simulink model "NeuromuscularModel2D"  (R2019b)
settings: Solver=ode15s  StartTime=0.0  StopTime=30  MaxStep=.01  RelTol=1e-4  AbsTol=1e-6  EnableMultiTasking=on
values from neighbouring files (symbols this model uses):
  dt_visual = 1/50    (= 0.02)    [evaluateCost.m]    (also in optimize.m = 0.0333333333333; setVars.m = 0.0333333333333)
  initialTargetAngle = 70*pi/180    (= 1.2217304764)    [ControlParams.m]    (also in setInit.m)
  LongDelay = 0.020/2    (= 0.01)    [ControlParams.m]
  LongLoopDelay = 0.030    (= 0.03)    [ControlParams.m]
  MidDelay = 0.010/2    (= 0.005)    [ControlParams.m]
  N = {S.name}    [mergeCompareEnergyCosts.m]
  PreStimBFSHst = 0.02    [ControlParams.m]    (also in assignGainsSagittal.m = GainsSagittal(51))
  PreStimBFSHsw = 0.02    [ControlParams.m]    (also in assignGainsSagittal.m = GainsSagittal(60))
  PreStimGASst = 0.01    [ControlParams.m]    (also in assignGainsSagittal.m = GainsSagittal(52))
  PreStimGASsw = 0.01    [ControlParams.m]    (also in assignGainsSagittal.m = GainsSagittal(61))
  PreStimGLUst = 0.05    [ControlParams.m]    (also in assignGainsSagittal.m = GainsSagittal(47))
  PreStimGLUsw = 0.01    [ControlParams.m]    (also in assignGainsSagittal.m = GainsSagittal(56))
  PreStimHAMst = 0.05    [ControlParams.m]    (also in assignGainsSagittal.m = GainsSagittal(48))
  PreStimHAMsw = 0.01    [ControlParams.m]    (also in assignGainsSagittal.m = GainsSagittal(57))
  PreStimHFLst = 0.05    [ControlParams.m]    (also in assignGainsSagittal.m = GainsSagittal(46))
  PreStimHFLsw = 0.01    [ControlParams.m]    (also in assignGainsSagittal.m = GainsSagittal(55))
  PreStimRFst = 0.01    [ControlParams.m]    (also in assignGainsSagittal.m = GainsSagittal(49))
  PreStimRFsw = 0.01    [ControlParams.m]    (also in assignGainsSagittal.m = GainsSagittal(58))
  PreStimSOLst = 0.01    [ControlParams.m]    (also in assignGainsSagittal.m = GainsSagittal(53))
  PreStimSOLsw = 0.01    [ControlParams.m]    (also in assignGainsSagittal.m = GainsSagittal(62))
  PreStimTAst = 0.01    [ControlParams.m]    (also in assignGainsSagittal.m = GainsSagittal(54))
  PreStimTAsw = 0.01    [ControlParams.m]    (also in assignGainsSagittal.m = GainsSagittal(63))
  PreStimVASst = 0.08    [ControlParams.m]    (also in assignGainsSagittal.m = GainsSagittal(50))
  PreStimVASsw = 0.01    [ControlParams.m]    (also in assignGainsSagittal.m = GainsSagittal(59))
  ShortDelay = 0.005/2    (= 0.0025)    [ControlParams.m]
  termination_height = 0.5    [ControlParams.m]
  X = ~cellfun('isempty',strfind(N,'compareEnergyCost'))    [mergeCompareEnergyCosts.m]
undefined symbols (not defined in the file or in its folder): g, hatLeftHipToCenterDistWidth, hatLeftHipToCG, initialTargetAngleR, magnitude, obstacle_depth, obstacle_height, obstacle_width, obstacle_x, PreStimHABst, PreStimHABsw, PreStimHADst, PreStimHADsw, thetaHATref, Y, Z
libraries: NeuroMuscularLibrary x96, sm_lib x20, nesl_utility x19, simulink x3
(part 3 of 3)

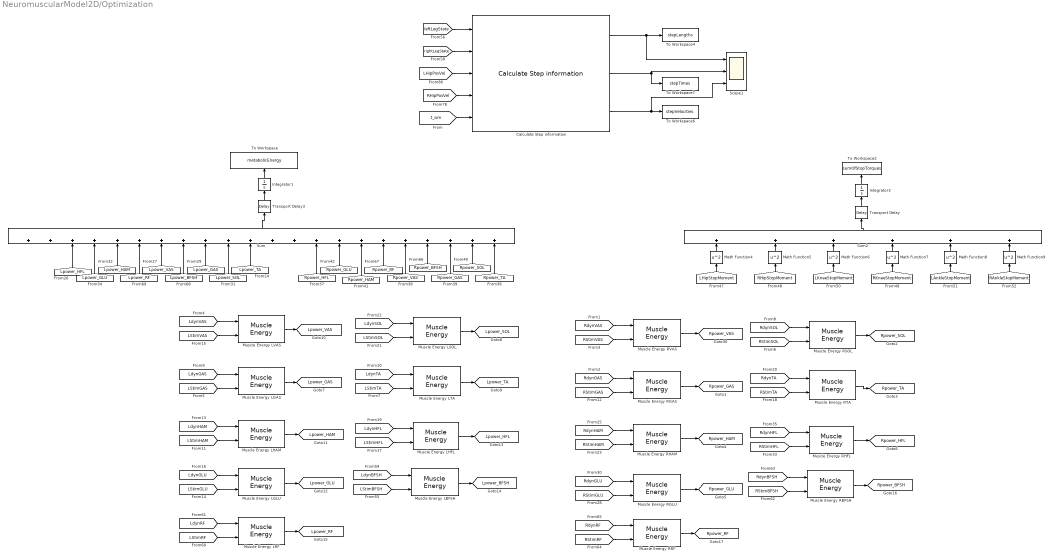
== system NeuromuscularModel2D/Optimization ==
  Calculate Step information : NeuroMuscularLibrary/Calculate Step information  SystemSampleTime=-1  Latency=0  AutoFrameSizeCalculation=off
  Integrator1 : Integrator
  Integrator3 : Integrator
  Math Function{4..9} (6 alike) : Math  Operator=square  SaturateOnIntegerOverflow=on
  Muscle Energy LBFSH : NeuroMuscularLibrary/Muscle Energy  lopt=loptBFSH  FT=FT_BFSH  Fmax=FmaxBFSH  vmax=vmaxBFSH
  Muscle Energy LGAS : NeuroMuscularLibrary/Muscle Energy  lopt=loptGAS  FT=FT_GAS  Fmax=FmaxGAS  vmax=vmaxGAS
  Muscle Energy LGLU : NeuroMuscularLibrary/Muscle Energy  lopt=loptGLU  FT=FT_GLU  Fmax=FmaxGLU  vmax=vmaxGLU
  Muscle Energy LHAM : NeuroMuscularLibrary/Muscle Energy  lopt=loptHAM  FT=FT_HAM  Fmax=FmaxHAM  vmax=vmaxHAM
  Muscle Energy LHFL : NeuroMuscularLibrary/Muscle Energy  lopt=loptHFL  FT=FT_HFL  Fmax=FmaxHFL  vmax=vmaxHFL
  Muscle Energy LRF : NeuroMuscularLibrary/Muscle Energy  lopt=loptRF  FT=FT_RF  Fmax=FmaxRF  vmax=vmaxRF
  Muscle Energy LSOL : NeuroMuscularLibrary/Muscle Energy  lopt=loptSOL  FT=FT_SOL  Fmax=FmaxSOL  vmax=vmaxSOL
  Muscle Energy LTA : NeuroMuscularLibrary/Muscle Energy  lopt=loptTA  FT=FT_TA  Fmax=FmaxTA  vmax=vmaxTA
  Muscle Energy LVAS : NeuroMuscularLibrary/Muscle Energy  lopt=loptVAS  FT=FT_VAS  Fmax=FmaxVAS  vmax=vmaxVAS
  Muscle Energy RBFSH : NeuroMuscularLibrary/Muscle Energy  lopt=loptBFSH  FT=FT_BFSH  Fmax=FmaxBFSH  vmax=vmaxBFSH
  Muscle Energy RGAS : NeuroMuscularLibrary/Muscle Energy  lopt=loptGAS  FT=FT_GAS  Fmax=FmaxGAS  vmax=vmaxGAS
  Muscle Energy RGLU : NeuroMuscularLibrary/Muscle Energy  lopt=loptGLU  FT=FT_GLU  Fmax=FmaxGLU  vmax=vmaxGLU
  Muscle Energy RHAM : NeuroMuscularLibrary/Muscle Energy  lopt=loptHAM  FT=FT_HAM  Fmax=FmaxHAM  vmax=vmaxHAM
  Muscle Energy RHFL : NeuroMuscularLibrary/Muscle Energy  lopt=loptHFL  FT=FT_HFL  Fmax=FmaxHFL  vmax=vmaxHFL
  Muscle Energy RRF : NeuroMuscularLibrary/Muscle Energy  lopt=loptRF  FT=FT_RF  Fmax=FmaxRF  vmax=vmaxRF
  Muscle Energy RSOL : NeuroMuscularLibrary/Muscle Energy  lopt=loptSOL  FT=FT_SOL  Fmax=FmaxSOL  vmax=vmaxSOL
  Muscle Energy RTA : NeuroMuscularLibrary/Muscle Energy  lopt=loptTA  FT=FT_TA  Fmax=FmaxTA  vmax=vmaxTA
  Muscle Energy RVAS : NeuroMuscularLibrary/Muscle Energy  lopt=loptVAS  FT=FT_VAS  Fmax=FmaxVAS  vmax=vmaxVAS
  Scope1 : Scope  NumInputPorts=3
  Sum : Sum  Inputs=++++++++++++++++++++++
  Sum2 : Sum  Inputs=++++++
  To Workspace : ToWorkspace  VariableName=metabolicEnergy  SampleTime=-1
      settings: MaxDataPoints=1
  To Workspace2 : ToWorkspace  VariableName=sumOfStopTorques  SampleTime=-1
      settings: MaxDataPoints=1
  To Workspace4 : ToWorkspace  VariableName=stepLengths  SampleTime=-1
  To Workspace6 : ToWorkspace  VariableName=stepVelocities  SampleTime=-1
  To Workspace7 : ToWorkspace  VariableName=stepTimes  SampleTime=-1
  Transport Delay : TransportDelay  DelayTime=3  BufferSize=24576
  Transport Delay3 : TransportDelay  DelayTime=3  BufferSize=24576
  tag scope: Lpower_BFSH=global, Lpower_GAS=global, Lpower_GLU=global, Lpower_HAM=global, Lpower_HFL=global, Lpower_RF=global, Lpower_SOL=global, Lpower_TA=global, Lpower_VAS=global, Rpower_BFSH=global, Rpower_GAS=global, Rpower_GLU=global, Rpower_HAM=global, Rpower_HFL=global, Rpower_RF=global, Rpower_SOL=global, Rpower_TA=global, Rpower_VAS=global
  wires:
  [RdynSOL] -> Muscle Energy RSOL/1
  [RStimSOL] -> Muscle Energy RSOL/2
  [RStimVAS] -> Muscle Energy RVAS/2
  [RStimGAS] -> Muscle Energy RGAS/2
  Muscle Energy RVAS/1 -> [Rpower_VAS]
  Muscle Energy RGAS/1 -> [Rpower_GAS]
  Muscle Energy RSOL/1 -> [Rpower_SOL]
  Muscle Energy RTA/1 -> [Rpower_TA]
  [RdynTA] -> Muscle Energy RTA/1
  [RStimTA] -> Muscle Energy RTA/2
  [RdynHAM] -> Muscle Energy RHAM/1
  [RStimHAM] -> Muscle Energy RHAM/2
  [RdynGLU] -> Muscle Energy RGLU/1
  [RStimGLU] -> Muscle Energy RGLU/2
  [RdynHFL] -> Muscle Energy RHFL/1
  [RStimHFL] -> Muscle Energy RHFL/2
  Muscle Energy RHAM/1 -> [Rpower_HAM]
  Muscle Energy RGLU/1 -> [Rpower_GLU]
  Muscle Energy RHFL/1 -> [Rpower_HFL]
  [Lpower_VAS] -> Sum/7
  [Lpower_RF] -> Sum/6
  [Lpower_HAM] -> Sum/5
  [Lpower_GLU] -> Sum/4
  [Lpower_HFL] -> Sum/3
  [RdynGAS] -> Muscle Energy RGAS/1
  [RdynVAS] -> Muscle Energy RVAS/1
  [LdynSOL] -> Muscle Energy LSOL/1
  [LStimSOL] -> Muscle Energy LSOL/2
  [LStimVAS] -> Muscle Energy LVAS/2
  [LStimGAS] -> Muscle Energy LGAS/2
  Muscle Energy LVAS/1 -> [Lpower_VAS]
  Muscle Energy LGAS/1 -> [Lpower_GAS]
  Muscle Energy LSOL/1 -> [Lpower_SOL]
  Muscle Energy LTA/1 -> [Lpower_TA]
  [LdynTA] -> Muscle Energy LTA/1
  [LStimTA] -> Muscle Energy LTA/2
  [LdynHAM] -> Muscle Energy LHAM/1
  [LStimHAM] -> Muscle Energy LHAM/2
  [LdynGLU] -> Muscle Energy LGLU/1
  [LStimGLU] -> Muscle Energy LGLU/2
  [LdynHFL] -> Muscle Energy LHFL/1
  [LStimHFL] -> Muscle Energy LHFL/2
  Muscle Energy LHAM/1 -> [Lpower_HAM]
  Muscle Energy LGLU/1 -> [Lpower_GLU]
  Muscle Energy LHFL/1 -> [Lpower_HFL]
  [LdynGAS] -> Muscle Energy LGAS/1
  [LdynVAS] -> Muscle Energy LVAS/1
  [Lpower_SOL] -> Sum/10
  [Rpower_HAM] -> Sum/16
  [Rpower_GLU] -> Sum/15
  [Rpower_HFL] -> Sum/14
  [Lpower_TA] -> Sum/11
  Integrator1/1 -> To Workspace/1
  Sum/1 -> Transport Delay3/1
  Integrator3/1 -> To Workspace2/1
  Math Function4/1 -> Sum2/1
  [LHipStopMoment] -> Math Function4/1
  Math Function5/1 -> Sum2/2
  [RHipStopMoment] -> Math Function5/1
  Math Function6/1 -> Sum2/3
  Math Function7/1 -> Sum2/4
  [LKneeStopMoment] -> Math Function6/1
  [RKneeStopMoment] -> Math Function7/1
  [LAnkleStopMoment] -> Math Function8/1
  Math Function8/1 -> Sum2/5
  [RAnkleStopMoment] -> Math Function9/1
  Math Function9/1 -> Sum2/6
  Transport Delay/1 -> Integrator3/1
  Sum2/1 -> Transport Delay/1
  Transport Delay3/1 -> Integrator1/1
  [rightLegState] -> Calculate Step information/2
  Calculate Step information/1 -> Scope1/1, To Workspace4/1
  Calculate Step information/3 -> To Workspace6/1, Scope1/3
  Calculate Step information/2 -> To Workspace7/1, Scope1/2
  [leftLegState] -> Calculate Step information/1
  [t_sim] -> Calculate Step information/5
  Muscle Energy LBFSH/1 -> [Lpower_BFSH]
  [LStimBFSH] -> Muscle Energy LBFSH/2
  [LdynBFSH] -> Muscle Energy LBFSH/1
  [LdynRF] -> Muscle Energy LRF/1
  [LStimRF] -> Muscle Energy LRF/2
  Muscle Energy LRF/1 -> [Lpower_RF]
  Muscle Energy RRF/1 -> [Rpower_RF]
  [RdynRF] -> Muscle Energy RRF/1
  Muscle Energy RBFSH/1 -> [Rpower_BFSH]
  [RStimRF] -> Muscle Energy RRF/2
  [RStimBFSH] -> Muscle Energy RBFSH/2
  [RdynBFSH] -> Muscle Energy RBFSH/1
  [Lpower_BFSH] -> Sum/8
  [Lpower_GAS] -> Sum/9
  [Rpower_VAS] -> Sum/18
  [Rpower_RF] -> Sum/17
  [Rpower_TA] -> Sum/22
  [Rpower_SOL] -> Sum/21
  [Rpower_GAS] -> Sum/20
  [Rpower_BFSH] -> Sum/19
  [RHipPosVel] -> Calculate Step information/4
  [LHipPosVel] -> Calculate Step information/3

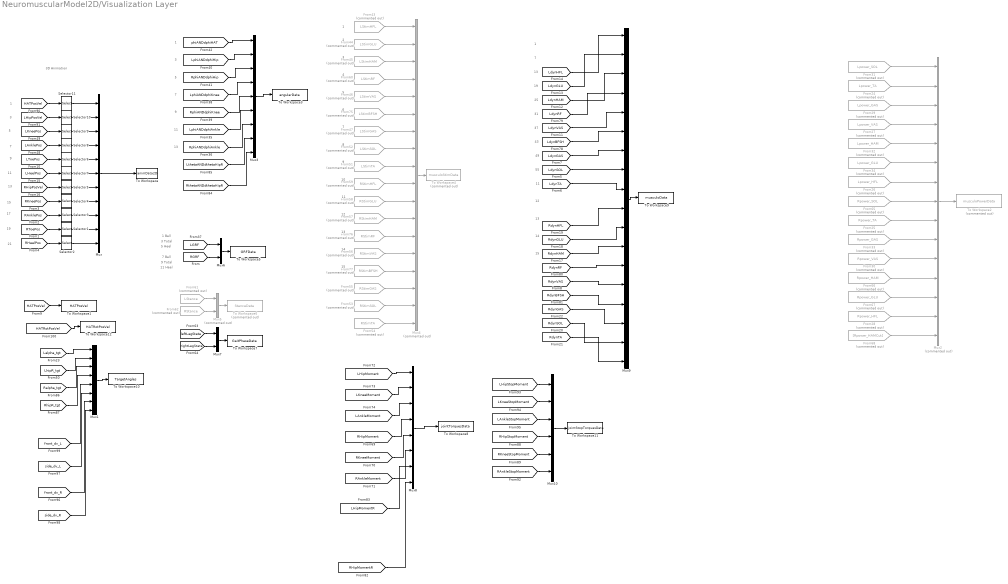
== system NeuromuscularModel2D/Visualization Layer ==
  note: 21
  note: 19
  note: 17
  note: 15
  note: 13
  note: 11
  note: 9
  note: 7
  note: 5
  note: 3
  note: 1
  note: 3D Animation
  note: 1
  note: 8
  note: 13
  note: 3
  note: 1
  note: 5
  note: 10
  note: 4
  note: 6
  note: 3
  note: 5
  note: 7
  note: 9
  note: 9
  note: 11
  note: 2
  note: 7
  note: 11
  note: 12
  note: 15
  note: 9 Total
  note: 1 Ball
  note: 5 Heel
  note: 14
  note: 11 Heel
  note: 3 Total
  note: 13
  note: 7 Ball
  note: 7
  note: 12
  note: 13
  note: 55
  note: 14
  note: 19
  note: 1
  note: 43
  note: 49
  note: 37
  note: 25
  note: 11
  note: 13
  note: 15
  note: 31
  From24 : From  Commented=on  GotoTag=Lpower_TA  TagVisibility=global
  From25 : From  Commented=on  GotoTag=Rpower_TA  TagVisibility=global
  From26 : From  Commented=on  GotoTag=Lpower_HFL  TagVisibility=global
  From27 : From  Commented=on  GotoTag=Lpower_VAS  TagVisibility=global
  From28 : From  Commented=on  GotoTag=Rpower_HFL  TagVisibility=global
  From29 : From  Commented=on  GotoTag=Lpower_GAS  TagVisibility=global
  From30 : From  Commented=on  GotoTag=Rpower_VAS  TagVisibility=global
  From31 : From  Commented=on  GotoTag=Lpower_SOL  TagVisibility=global
  From32 : From  Commented=on  GotoTag=Lpower_HAM  TagVisibility=global
  From33 : From  Commented=on  GotoTag=Rpower_GAS  TagVisibility=global
  From34 : From  Commented=on  GotoTag=Lpower_GLU  TagVisibility=global
  From43 : From  Commented=on  GotoTag=LStimHFL  TagVisibility=global
  From44 : From  Commented=on  GotoTag=LStimGLU  TagVisibility=global
  From45 : From  Commented=on  GotoTag=LStimHAM  TagVisibility=global
  From46 : From  Commented=on  GotoTag=LStimVAS  TagVisibility=global
  From47 : From  Commented=on  GotoTag=LStimGAS  TagVisibility=global
  From51 : From  Commented=on  GotoTag=LStimTA  TagVisibility=global
  From52 : From  Commented=on  GotoTag=LStimSOL  TagVisibility=global
  From53 : From  Commented=on  GotoTag=RStimSOL  TagVisibility=global
  From54 : From  Commented=on  GotoTag=RStimTA  TagVisibility=global
  From55 : From  Commented=on  GotoTag=RStimGAS  TagVisibility=global
  From56 : From  Commented=on  GotoTag=RStimVAS  TagVisibility=global
  From57 : From  Commented=on  GotoTag=RStimHAM  TagVisibility=global
  From58 : From  Commented=on  GotoTag=RStimGLU  TagVisibility=global
  From59 : From  Commented=on  GotoTag=RStimHFL  TagVisibility=global
  From60 : From  Commented=on  GotoTag=LStimRF  TagVisibility=global
  From61 : From  Commented=on  GotoTag=LStance  TagVisibility=global
  From62 : From  Commented=on  GotoTag=RStance  TagVisibility=global
  From65 : From  Commented=on  GotoTag=Rpower_SOL  TagVisibility=global
  From66 : From  Commented=on  GotoTag=Rpower_HAM  TagVisibility=global
  From67 : From  Commented=on  GotoTag=Rpower_GLU  TagVisibility=global
  From68 : From  Commented=on  GotoTag=Rpower_HAMCut
  From75 : From  Commented=on  GotoTag=LStimBFSH  TagVisibility=global
  From76 : From  Commented=on  GotoTag=RStimRF  TagVisibility=global
  From77 : From  Commented=on  GotoTag=RStimBFSH  TagVisibility=global
  Mux : Mux  Inputs=11
  Mux1 : Mux  Inputs=8
  Mux10 : Mux  Inputs=6
  Mux2 : Mux  Commented=on  Inputs=15
  Mux3 : Mux  Inputs=9
  Mux4 : Mux  Commented=on  Inputs=18
  Mux5 : Mux  Commented=on  Inputs=2
  Mux6 : Mux  Inputs=2
  Mux7 : Mux  Inputs=2
  Mux8 : Mux  Inputs=8
  Mux9 : Mux  Inputs=18
  Selector{1..4,6..9} (8 alike) : Selector  InputPortWidth=3  IndexOptions=Index vector (dialog)  Indices=[1 3]  OutputSizes=1
  Selector10 : Selector  InputPortWidth=6  IndexOptions=Index vector (dialog)  Indices=[1 3]  OutputSizes=1
  Selector11 : Selector  InputPortWidth=6  IndexOptions=Index vector (dialog)  Indices=[1 3]  OutputSizes=1
  Selector5 : Selector  InputPortWidth=6  IndexOptions=Index vector (dialog)  Indices=[1 3]  OutputSizes=1
  To Workspace : ToWorkspace  VariableName=animData2D  SaveFormat=Structure With Time  SampleTime=1/30
  To Workspace1 : ToWorkspace  VariableName=HATPosVel  SaveFormat=Structure With Time  SampleTime=dt_visual
  To Workspace10 : ToWorkspace  VariableName=TargetAngles  SaveFormat=Structure With Time  SampleTime=dt_visual
  To Workspace11 : ToWorkspace  VariableName=jointStopTorquesData  SaveFormat=Structure With Time  SampleTime=dt_visual
  To Workspace12 : ToWorkspace  VariableName=HATRotPosVel  SaveFormat=Structure With Time  SampleTime=dt_visual
  To Workspace2 : ToWorkspace  Commented=on  VariableName=musculoPowerData  SaveFormat=Structure With Time  SampleTime=dt_visual
  To Workspace3 : ToWorkspace  VariableName=angularData  SaveFormat=Structure With Time  SampleTime=dt_visual
  To Workspace4 : ToWorkspace  Commented=on  VariableName=musculoStimData  SaveFormat=Structure With Time  SampleTime=dt_visual
  To Workspace5 : ToWorkspace  VariableName=GRFData  SaveFormat=Structure With Time  SampleTime=dt_visual
  To Workspace6 : ToWorkspace  Commented=on  VariableName=StanceData  SaveFormat=Structure With Time  SampleTime=1/30
  To Workspace7 : ToWorkspace  VariableName=GaitPhaseData  SaveFormat=Structure With Time  SampleTime=dt_visual
  To Workspace8 : ToWorkspace  VariableName=jointTorquesData  SaveFormat=Structure With Time  SampleTime=dt_visual
  To Workspace9 : ToWorkspace  VariableName=musculoData  SaveFormat=Structure With Time  SampleTime=dt_visual
  wires:
  [RAnklePos] -> Selector3/1
  [RKneePos] -> Selector4/1
  [RHipPosVel] -> Selector5/1
  [HATPosVel] -> Selector11/1
  [LHeelPos] -> Selector7/1
  [LToePos] -> Selector6/1
  [LAnklePos] -> Selector8/1
  [LKneePos] -> Selector9/1
  [LHipPosVel] -> Selector10/1
  Selector11/1 -> Mux/1
  Selector3/1 -> Mux/9
  Selector4/1 -> Mux/8
  Selector5/1 -> Mux/7
  Selector7/1 -> Mux/6
  Selector6/1 -> Mux/5
  Selector8/1 -> Mux/4
  Selector9/1 -> Mux/3
  Selector10/1 -> Mux/2
  Mux/1 -> To Workspace/1
  [RHeelPos] -> Selector2/1
  [RToePos] -> Selector1/1
  Selector2/1 -> Mux/11
  Selector1/1 -> Mux/10
  From61/1 -> Mux5/1
  From75/1 -> Mux4/6
  Mux4/1 -> To Workspace4/1
  [RphiANDdphiAnkle] -> Mux3/7
  Mux5/1 -> To Workspace6/1
  Mux6/1 -> To Workspace5/1
  From76/1 -> Mux4/13
  [RGRF] -> Mux6/2
  [phiANDdphiHAT] -> Mux3/1
  From51/1 -> Mux4/9
  Mux3/1 -> To Workspace3/1
  [LphiANDdphiAnkle] -> Mux3/6
  From58/1 -> Mux4/11
  [LphiANDdphiKnee] -> Mux3/4
  From57/1 -> Mux4/12
  From77/1 -> Mux4/15
  [LGRF] -> Mux6/1
  From56/1 -> Mux4/14
  [LphiANDdphiHip] -> Mux3/2
  From52/1 -> Mux4/8
  [RphiANDdphiKnee] -> Mux3/5
  From45/1 -> Mux4/3
  From43/1 -> Mux4/1
  From46/1 -> Mux4/5
  From59/1 -> Mux4/10
  From47/1 -> Mux4/7
  From44/1 -> Mux4/2
  From62/1 -> Mux5/2
  [RphiANDdphiHip] -> Mux3/3
  From60/1 -> Mux4/4
  [rightLegState] -> Mux7/2
  Mux7/1 -> To Workspace7/1
  [leftLegState] -> Mux7/1
  From31/1 -> Mux2/1
  From24/1 -> Mux2/2
  From29/1 -> Mux2/3
  From27/1 -> Mux2/4
  From32/1 -> Mux2/5
  From34/1 -> Mux2/6
  From26/1 -> Mux2/7
  From65/1 -> Mux2/8
  From25/1 -> Mux2/9
  From33/1 -> Mux2/10
  From30/1 -> Mux2/11
  From66/1 -> Mux2/12
  From67/1 -> Mux2/13
  From28/1 -> Mux2/14
  From68/1 -> Mux2/15
  Mux2/1 -> To Workspace2/1
  Mux8/1 -> To Workspace8/1
  [LHipMoment] -> Mux8/1
  [LKneeMoment] -> Mux8/2
  [LAnkleMoment] -> Mux8/3
  [RHipMoment] -> Mux8/4
  [RKneeMoment] -> Mux8/5
  [RAnkleMoment] -> Mux8/6
  From55/1 -> Mux4/16
  From53/1 -> Mux4/17
  From54/1 -> Mux4/18
  Mux9/1 -> To Workspace9/1
  [RdynHAM] -> Mux9/12
  [LdynHFL] -> Mux9/1
  [RdynGLU] -> Mux9/11
  [RdynVAS] -> Mux9/14
  [LdynBFSH] -> Mux9/6
  [RdynGAS] -> Mux9/16
  [RdynBFSH] -> Mux9/15
  [LdynVAS] -> Mux9/5
  [LdynGAS] -> Mux9/7
  [LdynSOL] -> Mux9/8
  [LdynRF] -> Mux9/4
  [LdynHAM] -> Mux9/3
  [LdynGLU] -> Mux9/2
  [LdynTA] -> Mux9/9
  [RdynRF] -> Mux9/13
  [RdynHFL] -> Mux9/10
  [RdynSOL] -> Mux9/17
  [RdynTA] -> Mux9/18
  [LHipMomentR] -> Mux8/7
  [RHipMomentR] -> Mux8/8
  [LthetaANDdthetaHipR] -> Mux3/8
  [RthetaANDdthetaHipR] -> Mux3/9
  [HATPosVel] -> To Workspace1/1
  [LHipStopMoment] -> Mux10/1
  [LKneeStopMoment] -> Mux10/2
  [LAnkleStopMoment] -> Mux10/3
  [RHipStopMoment] -> Mux10/4
  [RKneeStopMoment] -> Mux10/5
  [RAnkleStopMoment] -> Mux10/6
  Mux10/1 -> To Workspace11/1
  [Lalpha_tgt] -> Mux1/1
  [front_dv_R] -> Mux1/7
  [side_dv_R] -> Mux1/8
  [LhipR_tgt] -> Mux1/2
  [side_dv_L] -> Mux1/6
  [front_dv_L] -> Mux1/5
  [Ralpha_tgt] -> Mux1/3
  Mux1/1 -> To Workspace10/1
  [RhipR_tgt] -> Mux1/4
  [HATRotPosVel] -> To Workspace12/1

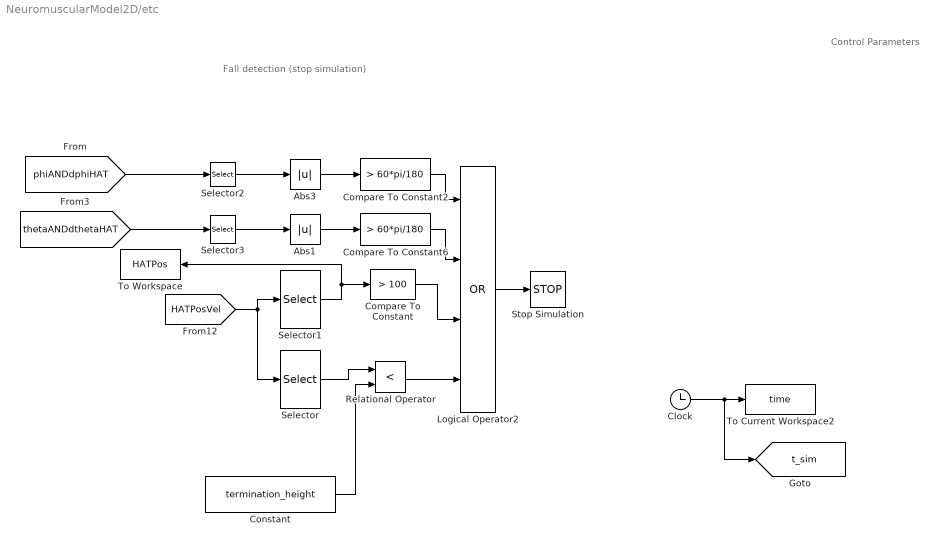
== system NeuromuscularModel2D/etc ==
  note: Fall detection
      | (stop simulation)
  note: Control Parameters
  Abs1 : Abs
  Abs3 : Abs
  Clock : Clock
  Compare To Constant : simulink/Logic and Bit Operations/Compare To Constant  relop=>  const=100  OutDataTypeStr=boolean
  Compare To Constant2 : simulink/Logic and Bit Operations/Compare To Constant  relop=>  const=60*pi/180  OutDataTypeStr=boolean
  Compare To Constant6 : simulink/Logic and Bit Operations/Compare To Constant  relop=>  const=60*pi/180  OutDataTypeStr=boolean
  Constant : Constant  Value=termination_height
  Logical Operator2 : Logic  Operator=OR  Inputs=4  AllPortsSameDT=off  OutDataTypeStr=boolean
  Relational Operator : RelationalOperator  Operator=<  OutDataTypeStr=boolean  RndMeth=Nearest
  Selector : Selector  InputPortWidth=6  IndexOptions=Index vector (dialog)  Indices=[3]  OutputSizes=1
  Selector1 : Selector  InputPortWidth=6  IndexOptions=Index vector (dialog)  Indices=[1]  OutputSizes=1
  Selector2 : Selector  InputPortWidth=2  IndexOptions=Index vector (dialog)  Indices=[1]  OutputSizes=1
  Selector3 : Selector  InputPortWidth=2  IndexOptions=Index vector (dialog)  Indices=[1]  OutputSizes=1
  Stop Simulation : Stop
  To Current Workspace2 : ToWorkspace  VariableName=time  SampleTime=-1
      settings: MaxDataPoints=1
  To Workspace : ToWorkspace  VariableName=HATPos  SampleTime=-1
      settings: MaxDataPoints=1
  tag scope: t_sim=global
  wires:
  Selector2/1 -> Abs3/1
  Abs3/1 -> Compare To Constant2/1
  Compare To Constant2/1 -> Logical Operator2/1
  Logical Operator2/1 -> Stop Simulation/1
  Selector3/1 -> Abs1/1
  Abs1/1 -> Compare To Constant6/1
  Compare To Constant6/1 -> Logical Operator2/2
  Compare To Constant/1 -> Logical Operator2/3
  Selector/1 -> Relational Operator/1
  Selector1/1 -> Compare To Constant/1, To Workspace/1
  Constant/1 -> Relational Operator/2
  Relational Operator/1 -> Logical Operator2/4
  [HATPosVel] -> Selector/1, Selector1/1
  Clock/1 -> [t_sim], To Current Workspace2/1
  [phiANDdphiHAT] -> Selector2/1
  [thetaANDdthetaHAT] -> Selector3/1

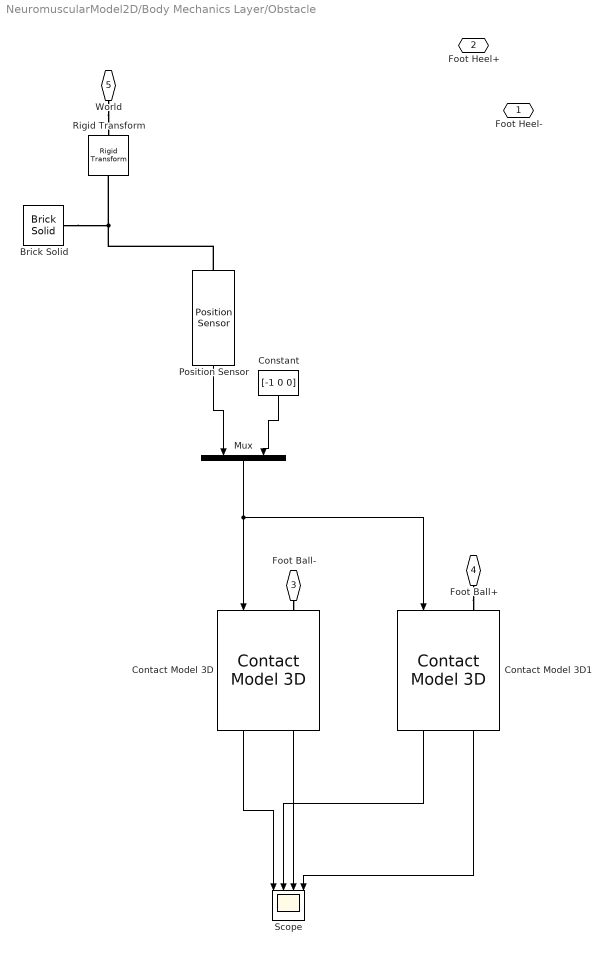
== system NeuromuscularModel2D/Body Mechanics Layer/Obstacle ==
  Brick Solid : sm_lib/Body Elements/Brick Solid  GraphicAmbientColor=[0.15 0.15 0.15 1.0]  BasedOnType=Mass  BrickDimensions=[obstacle_depth obstacle_height obstacle_width]  BrickDimensionUnits=m  CenterOfMass=[0 0 0]  CenterOfMassUnits=m  GraphicDiffuseColor=[0.6 1.0 0.2]  Density=1000  DensityUnits=kg/m^3  DoExposeReferenceFrame=on  GraphicEmissiveColor=[0.0 0.0 0.0 1.0]  ExportEntireGeometry=off  SerializedFrames=<Frames/>  MarkerShape=Sphere  MarkerSize=10  GraphicType=FromGeometry  InertiaType=CalculateFromGeometry  Mass=0  MassUnits=kg  MomentsOfInertia=[1 1 1]  MomentsOfInertiaUnits=kg*m^2  GraphicOpacity=1.0  ProductsOfInertia=[0 0 0]  ProductsOfInertiaUnits=kg*m^2  GraphicShininess=75  GraphicSpecularColor=[0.5 0.5 0.5 1.0]  GraphicVisPropType=SimpleVisualProperties
  Constant : Constant  Value=[-1 0 0]
  Contact Model 3D : NeuroMuscularLibrary/Contact Model 3D  SystemSampleTime=-1  Latency=0  AutoFrameSizeCalculation=off
  Contact Model 3D1 : NeuroMuscularLibrary/Contact Model 3D  SystemSampleTime=-1  Latency=0  AutoFrameSizeCalculation=off
  Mux : Mux  Inputs=[3 3]
  Position Sensor : NeuroMuscularLibrary/Position Sensor  SystemSampleTime=-1  Latency=0  AutoFrameSizeCalculation=off
  Rigid Transform : sm_lib/Frames and Transforms/Rigid Transform  TranslationMethod=Cartesian  TranslationStandardOffset=0  TranslationLengthUnit=m  TranslationStandardAxis=+Z  TranslationCartesianOffset=[(obstacle_x+obstacle_depth/2) obstacle_height/2 0]  TranslationROffset=0  TranslationROffsetUnits=m  TranslationZOffset=0  TranslationZOffsetUnits=m  TranslationThetaOffset=0  TranslationThetaOffsetUnits=deg  RotationMethod=None  RotationAngleUnits=deg  RotationStandardAxis=+Z  RotationAngle=0.0  RotationArbitraryAxis=[0 0 1]  FollAlignAxisA=+X  BaseAlignAxisA=+Y  FollAlignAxisB=+Y  BaseAlignAxisB=+Z  RotationSequenceAxes=FollowerAxes  RotationSequence=XYX  RotationSequenceAngles=[0 0 0]  RotationSequenceAnglesUnits=deg  RotationMatrix=[1 0 0; 0 1 0; 0 0 1]
  Scope : Scope  NumInputPorts=4
  Foot Heel- : PMIOPort  Side=Left
  Foot Heel+ : PMIOPort  Port=2  Side=Left
  Foot Ball- : PMIOPort  Port=3  Side=Left
  Foot Ball+ : PMIOPort  Port=4  Side=Left
  World : PMIOPort  Port=5  Side=Left
  wires:
  Mux/1 -> Contact Model 3D1/1, Contact Model 3D/1
  Position Sensor/1 -> Mux/1
  Constant/1 -> Mux/2
  Contact Model 3D/2 -> Scope/3
  Contact Model 3D1/2 -> Scope/4
  Contact Model 3D1/1 -> Scope/2
  Contact Model 3D/1 -> Scope/1
  connections:
  Brick Solid/RConn1 -- Rigid Transform/RConn1 -- Position Sensor/LConn1
  Foot Ball-/RConn1 -- Contact Model 3D/LConn1
  World/RConn1 -- Rigid Transform/LConn1
  Foot Ball+/RConn1 -- Contact Model 3D1/LConn1

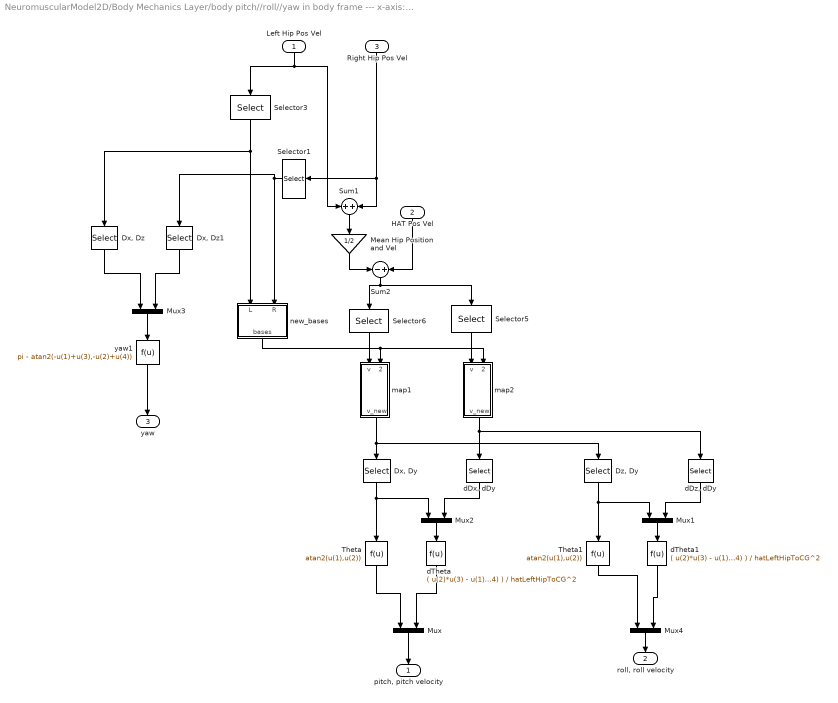
== system NeuromuscularModel2D/Body Mechanics Layer/body pitch//roll//yaw in body frame --- x-axis: forward y-axis: leftward z-axis: parallel to gravity ==
  Left Hip Pos Vel : Inport
  HAT Pos Vel : Inport  Port=2
  Right Hip Pos Vel : Inport  Port=3
  "Dx, Dy" : Selector  InputPortWidth=3  IndexOptions=Index vector (dialog)  Indices=[1 2]  OutputSizes=1
  "Dx, Dz" : Selector  InputPortWidth=3  IndexOptions=Index vector (dialog)  Indices=[1 2]  OutputSizes=1
  "Dx, Dz1" : Selector  InputPortWidth=3  IndexOptions=Index vector (dialog)  Indices=[1 2]  OutputSizes=1
  "Dz, Dy" : Selector  InputPortWidth=3  IndexOptions=Index vector (dialog)  Indices=[3 2]  OutputSizes=1
  Mean Hip Position and Vel : Gain  Gain=1/2
  Mux{,1..4} (5 alike) : Mux  Inputs=2
  Selector1 : Selector  InputPortWidth=6  IndexOptions=Index vector (dialog)  Indices=[1 2 3]  OutputSizes=1
  Selector3 : Selector  InputPortWidth=6  IndexOptions=Index vector (dialog)  Indices=[1 2 3]  OutputSizes=1
  Selector5 : Selector  InputPortWidth=6  IndexOptions=Index vector (dialog)  Indices=[4 5 6]  OutputSizes=1
  Selector6 : Selector  InputPortWidth=6  IndexOptions=Index vector (dialog)  Indices=[1 2 3]  OutputSizes=1
  Sum1 : Sum
  Sum2 : Sum  Inputs=-+
  Theta : Fcn  Expr=atan2(u(1),u(2))
  Theta1 : Fcn  Expr=atan2(u(1),u(2))
  "dDx, dDy" : Selector  InputPortWidth=3  IndexOptions=Index vector (dialog)  Indices=[1 2]  OutputSizes=1
  "dDz, dDy" : Selector  InputPortWidth=3  IndexOptions=Index vector (dialog)  Indices=[3 2]  OutputSizes=1
  dTheta : Fcn  Expr=( u(2)*u(3) - u(1)*u(4) ) / hatLeftHipToCG^2
  dTheta1 : Fcn  Expr=( u(2)*u(3) - u(1)*u(4) ) / hatLeftHipToCG^2
  map1 : Subsystem
  map2 : Subsystem
  new_bases : Subsystem
  yaw1 : Fcn  Expr=pi - atan2(-u(1)+u(3),-u(2)+u(4))
  "pitch, pitch velocity" : Outport
  "roll, roll velocity" : Outport  Port=2
  yaw : Outport  Port=3
  wires:
  "dDx, dDy"/1 -> Mux2/2
  Mux2/1 -> dTheta/1
  HAT Pos Vel/1 -> Sum2/2
  "Dx, Dy"/1 -> Mux2/1, Theta/1
  Selector3/1 -> "Dx, Dz"/1, new_bases/1(L)
  Selector1/1 -> "Dx, Dz1"/1, new_bases/2(R)
  Theta/1 -> Mux/1
  dTheta/1 -> Mux/2
  Selector6/1 -> map1/1(v)
  map1/1(v_new) -> "Dx, Dy"/1, "Dz, Dy"/1
  new_bases/1(bases) -> map1/2(basis), map2/2(basis)
  Selector5/1 -> map2/1(v)
  map2/1(v_new) -> "dDx, dDy"/1, "dDz, dDy"/1
  "dDz, dDy"/1 -> Mux1/2
  Mux1/1 -> dTheta1/1
  "Dz, Dy"/1 -> Mux1/1, Theta1/1
  Theta1/1 -> Mux4/1
  dTheta1/1 -> Mux4/2
  "Dx, Dz"/1 -> Mux3/1
  "Dx, Dz1"/1 -> Mux3/2
  Mux3/1 -> yaw1/1
  yaw1/1 -> yaw/1
  Left Hip Pos Vel/1 -> Sum1/1, Selector3/1
  Mean Hip Position and Vel/1 -> Sum2/1
  Sum1/1 -> Mean Hip Position and Vel/1
  Sum2/1 -> Selector6/1, Selector5/1
  Mux/1 -> "pitch, pitch velocity"/1
  Mux4/1 -> "roll, roll velocity"/1
  Right Hip Pos Vel/1 -> Sum1/2, Selector1/1

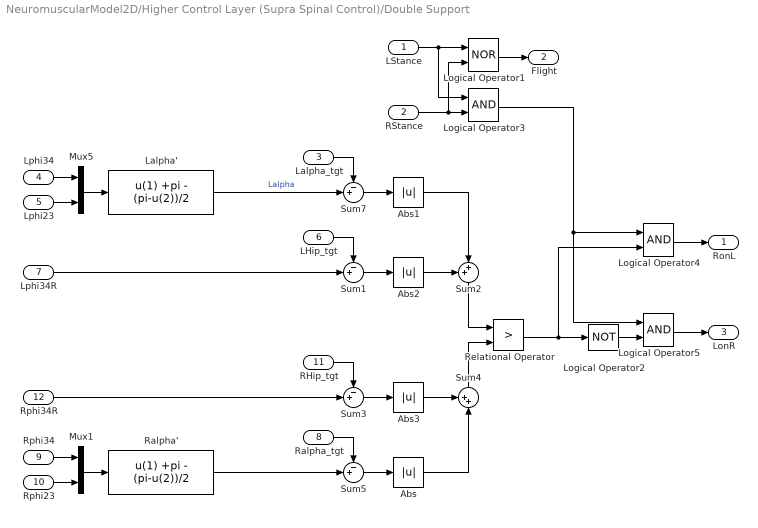
== system NeuromuscularModel2D/Higher Control Layer (Supra Spinal Control)/Double Support ==
  LStance : Inport
  RStance : Inport  Port=2
  Lalpha_tgt : Inport  Port=3
  Lphi34 : Inport  Port=4
  Lphi23 : Inport  Port=5
  LHip_tgt : Inport  Port=6
  Lphi34R : Inport  Port=7
  Ralpha_tgt : Inport  Port=8
  Rphi34 : Inport  Port=9
  Rphi23 : Inport  Port=10
  RHip_tgt : Inport  Port=11
  Rphi34R : Inport  Port=12
  Abs{,1..3} (4 alike) : Abs  ZeroCross=off
  Lalpha' : Fcn  Expr=u(1) +pi - (pi-u(2))/2
  Logical Operator1 : Logic  Operator=NOR  AllPortsSameDT=off  OutDataTypeStr=boolean
  Logical Operator2 : Logic  Operator=NOT  AllPortsSameDT=off
  Logical Operator3 : Logic  AllPortsSameDT=off
  Logical Operator4 : Logic  AllPortsSameDT=off
  Logical Operator5 : Logic  AllPortsSameDT=off
  Mux1 : Mux  Inputs=2
  Mux5 : Mux  Inputs=2
  Ralpha' : Fcn  Expr=u(1) +pi - (pi-u(2))/2
  Relational Operator : RelationalOperator  Operator=>  ZeroCross=off  RndMeth=Nearest
  Sum{1,3,5,7} (4 alike) : Sum  Inputs=-+|
  Sum2 : Sum  Inputs=++|
  Sum4 : Sum  Inputs=++|
  RonL : Outport
  Flight : Outport  Port=2
  LonR : Outport  Port=3
  wires:
  Lalpha'/1 -> Sum7/2  "Lalpha"
  Mux5/1 -> Lalpha'/1
  Ralpha'/1 -> Sum5/2
  Mux1/1 -> Ralpha'/1
  Sum5/1 -> Abs/1
  Sum7/1 -> Abs1/1
  LStance/1 -> Logical Operator3/1, Logical Operator1/1
  RStance/1 -> Logical Operator3/2, Logical Operator1/2
  Lalpha_tgt/1 -> Sum7/1
  Lphi34/1 -> Mux5/1
  Lphi23/1 -> Mux5/2
  Ralpha_tgt/1 -> Sum5/1
  Rphi34/1 -> Mux1/1
  Rphi23/1 -> Mux1/2
  Logical Operator1/1 -> Flight/1
  LHip_tgt/1 -> Sum1/1
  Lphi34R/1 -> Sum1/2
  Sum1/1 -> Abs2/1
  Abs2/1 -> Sum2/1
  Abs1/1 -> Sum2/2
  Sum2/1 -> Relational Operator/1
  RHip_tgt/1 -> Sum3/1
  Rphi34R/1 -> Sum3/2
  Sum3/1 -> Abs3/1
  Abs/1 -> Sum4/2
  Abs3/1 -> Sum4/1
  Sum4/1 -> Relational Operator/2
  Logical Operator4/1 -> RonL/1
  Logical Operator2/1 -> Logical Operator5/2
  Logical Operator5/1 -> LonR/1
  Relational Operator/1 -> Logical Operator2/1, Logical Operator4/2
  Logical Operator3/1 -> Logical Operator5/1, Logical Operator4/1

== system NeuromuscularModel2D/Body Mechanics Layer/body pitch//roll//yaw in body frame --- x-axis: forward y-axis: leftward z-axis: parallel to gravity/map1 ==
  v : Inport
  basis : Inport  Port=2
  Demux : Demux  Outputs=3
  Dot Product : DotProduct  InputSameDT=on  OutDataTypeStr=Inherit: Inherit via internal rule
  Dot Product1 : DotProduct  InputSameDT=on  OutDataTypeStr=Inherit: Inherit via internal rule
  Dot Product2 : DotProduct  InputSameDT=on  OutDataTypeStr=Inherit: Inherit via internal rule
  Mux3 : Mux  Inputs=3
  v_new : Outport
  wires:
  v/1 -> Dot Product2/2, Dot Product1/2, Dot Product/2
  Dot Product/1 -> Mux3/1
  Dot Product1/1 -> Mux3/2
  Dot Product2/1 -> Mux3/3
  Mux3/1 -> v_new/1  "v1"
  basis/1 -> Demux/1
  Demux/1 -> Dot Product/1
  Demux/2 -> Dot Product1/1
  Demux/3 -> Dot Product2/1

== system NeuromuscularModel2D/Body Mechanics Layer/body pitch//roll//yaw in body frame --- x-axis: forward y-axis: leftward z-axis: parallel to gravity/map2 ==
  v : Inport
  basis : Inport  Port=2
  Demux : Demux  Outputs=3
  Dot Product : DotProduct  InputSameDT=on  OutDataTypeStr=Inherit: Inherit via internal rule
  Dot Product1 : DotProduct  InputSameDT=on  OutDataTypeStr=Inherit: Inherit via internal rule
  Dot Product2 : DotProduct  InputSameDT=on  OutDataTypeStr=Inherit: Inherit via internal rule
  Mux3 : Mux  Inputs=3
  v_new : Outport
  wires:
  v/1 -> Dot Product2/2, Dot Product1/2, Dot Product/2
  Dot Product/1 -> Mux3/1
  Dot Product1/1 -> Mux3/2
  Dot Product2/1 -> Mux3/3
  Mux3/1 -> v_new/1  "v1"
  basis/1 -> Demux/1
  Demux/1 -> Dot Product/1
  Demux/2 -> Dot Product1/1
  Demux/3 -> Dot Product2/1

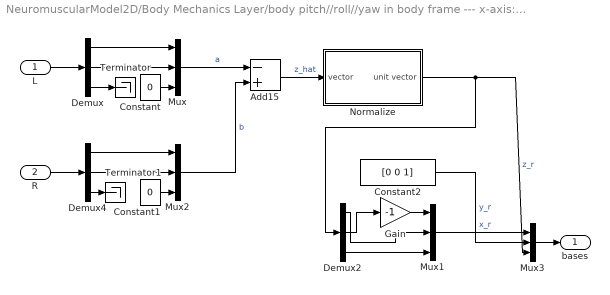
== system NeuromuscularModel2D/Body Mechanics Layer/body pitch//roll//yaw in body frame --- x-axis: forward y-axis: leftward z-axis: parallel to gravity/new_bases ==
  L : Inport
  R : Inport  Port=2
  Add15 : Sum  Inputs=-+
  Constant : Constant  Value=0
  Constant1 : Constant  Value=0
  Constant2 : Constant  Value=[0 0 1]
  Demux : Demux  Outputs=3
  Demux2 : Demux  Outputs=3
  Demux4 : Demux  Outputs=3
  Gain : Gain  Gain=-1
  Mux{,1..3} (4 alike) : Mux  Inputs=3
  Normalize : Subsystem
  Terminator : Terminator
  Terminator1 : Terminator
  bases : Outport
  wires:
  Constant2/1 -> Mux3/2  "y_r"
  Demux2/1 -> Mux1/2
  Demux2/3 -> Mux1/3
  Demux2/2 -> Gain/1
  Add15/1 -> Normalize/1(vector)  "z_hat"
  Normalize/1(unit vector) -> Demux2/1, Mux3/3  "z_r"
  Mux2/1 -> Add15/2  "b"
  Demux4/2 -> Mux2/2
  Constant1/1 -> Mux2/3
  Demux4/3 -> Terminator1/1
  Demux4/1 -> Mux2/1
  Mux/1 -> Add15/1  "a"
  Demux/2 -> Mux/2
  Constant/1 -> Mux/3
  Demux/3 -> Terminator/1
  Demux/1 -> Mux/1
  L/1 -> Demux/1
  R/1 -> Demux4/1
  Mux3/1 -> bases/1
  Gain/1 -> Mux1/1
  Mux1/1 -> Mux3/1  "x_r"

== system NeuromuscularModel2D/Body Mechanics Layer/body pitch//roll//yaw in body frame --- x-axis: forward y-axis: leftward z-axis: parallel to gravity/new_bases/Normalize ==
  vector : Inport
  Constant1 : Constant  Value=.5
  Math Function : Math  Operator=magnitude^2  SaturateOnIntegerOverflow=on
  Product : Product  Inputs=*/  RndMeth=Zero
  Sqrt : Math  Operator=pow  OutputSignalType=real  SaturateOnIntegerOverflow=on
  Sum of Elements : Sum  Inputs=+
  unit vector : Outport
  wires:
  Sqrt/1 -> Product/2
  Sum of Elements/1 -> Sqrt/1
  Math Function/1 -> Sum of Elements/1
  vector/1 -> Product/1, Math Function/1
  Product/1 -> unit vector/1  "x_r"
  Constant1/1 -> Sqrt/2
